simulink model "astrobee_control_sim"  (R2016b)
settings: configuration reference "cset" (kept outside this file)
PreLoadFcn:
  | astrobee_control_init;
  | astrobee_prep;
values from neighbouring files (symbols this model uses):
  astrobee_fsw_step_size = 0.016    [astrobee_control_init.m]    (also in astrobee_init.m)
  bus_cmc_msg_ic = Simulink.Bus.createMATLABStruct('cmc_msg')    [bus_init.m]
  bus_ctl_input_msg_ic = Simulink.Bus.createMATLABStruct('ctl_input_msg')    [bus_init.m]
undefined symbols (not defined in the file or in its folder): att_ki, att_kp, center_of_mass, cmc_mode_cmd, cmc_state_cmd_a, cmc_state_cmd_b, cmd_state_a, cmd_state_b, ctl_mode_cmd, current_time_nsec, current_time_sec, est_confidence, est_omega_B_ISS_B, est_P_B_ISS_ISS, est_quat_ISS2B, est_V_B_ISS_ISS, inertia_matrix, localization_mode_cmd, mass, omega_kd, pos_ki, pos_kp, speed_gain_cmd, tun_default_att_ki, tun_default_att_kp, tun_default_center_of_mass, tun_default_inertia_matrix, tun_default_mass, tun_default_omega_kd, tun_default_pos_ki, tun_default_pos_kp, tun_default_vel_kd, vel_kd
libraries: math_utils x3, cmc_command_and_mode_control x1, ctl_controller x1, env_environment_model_lib x1, fam_force_allocation_module_lib x1, simulink x1, veh_vehicle_model_lib x1
settings Model: Creator=mjmcinty  LastModifiedBy=jfusco1
settings ConfigSetRef: SourceLocation=Base Workspace

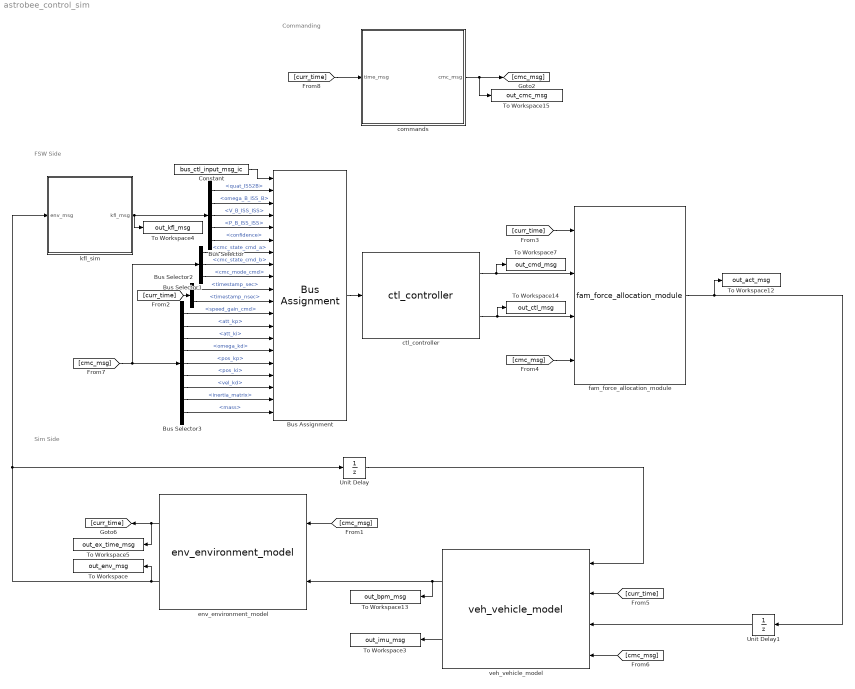
== system astrobee_control_sim ==
  note: FSW Side
  note: Sim Side
  note: Commanding
  Bus Assignment : BusAssignment  AssignedSignals=est_quat_ISS2B,est_omega_B_ISS_B,est_V_B_ISS_ISS,est_P_B_ISS_ISS,est_confidence,cmd_state_a,cmd_state_b,ctl_mode_cmd,current_time_sec,current_time_nsec,speed_gain_cmd,att_kp,att_ki,omega_kd,pos_kp,pos_ki,vel_kd,inertia_matrix,mass
  Bus Selector : BusSelector  OutputSignals=quat_ISS2B,omega_B_ISS_B,V_B_ISS_ISS,P_B_ISS_ISS,confidence
  Bus Selector1 : BusSelector  OutputSignals=cmc_state_cmd_a,cmc_state_cmd_b,cmc_mode_cmd
  Bus Selector2 : BusSelector  OutputSignals=timestamp_sec,timestamp_nsec
  Bus Selector3 : BusSelector  OutputSignals=speed_gain_cmd,att_kp,att_ki,omega_kd,pos_kp,pos_ki,vel_kd,inertia_matrix,mass
  Constant : Constant  Value=bus_ctl_input_msg_ic  OutDataTypeStr=Bus: ctl_input_msg
  To Workspace : ToWorkspace  VariableName=out_env_msg  SaveFormat=Timeseries  SampleTime=-1
  To Workspace12 : ToWorkspace  VariableName=out_act_msg  SaveFormat=Timeseries  SampleTime=-1
  To Workspace13 : ToWorkspace  VariableName=out_bpm_msg  SaveFormat=Timeseries  SampleTime=-1
  To Workspace14 : ToWorkspace  VariableName=out_ctl_msg  SaveFormat=Timeseries  SampleTime=-1
  To Workspace15 : ToWorkspace  VariableName=out_cmc_msg  SaveFormat=Timeseries  SampleTime=-1
  To Workspace3 : ToWorkspace  VariableName=out_imu_msg  SaveFormat=Timeseries  SampleTime=-1
  To Workspace4 : ToWorkspace  VariableName=out_kfl_msg  SaveFormat=Timeseries  SampleTime=-1
  To Workspace5 : ToWorkspace  VariableName=out_ex_time_msg  SaveFormat=Timeseries  SampleTime=-1
  To Workspace7 : ToWorkspace  VariableName=out_cmd_msg  SaveFormat=Timeseries  SampleTime=-1
  Unit Delay : UnitDelay  SampleTime=-1
  Unit Delay1 : UnitDelay  SampleTime=-1
  commands : Subsystem
  ctl_controller : ctl_controller/ctl_controller
  env_environment_model : env_environment_model_lib/env_environment_model  VariantControl=(default)
  fam_force_allocation_module : fam_force_allocation_module_lib/fam_force_allocation_module
  kfl_sim : Subsystem
  veh_vehicle_model : veh_vehicle_model_lib/veh_vehicle_model
  wires:
  [cmc_msg] -> fam_force_allocation_module/4
  env_environment_model/2 -> To Workspace/1, Unit Delay/1, kfl_sim/1(env_msg)
  ctl_controller/2 -> To Workspace14/1, fam_force_allocation_module/3
  ctl_controller/1 -> To Workspace7/1, fam_force_allocation_module/2
  [curr_time] -> fam_force_allocation_module/1
  commands/1(cmc_msg) -> To Workspace15/1, [cmc_msg]
  fam_force_allocation_module/1 -> To Workspace12/1, Unit Delay1/1
  [cmc_msg] -> env_environment_model/1
  [cmc_msg] -> veh_vehicle_model/4
  kfl_sim/1(kfl_msg) -> To Workspace4/1, Bus Selector/1
  veh_vehicle_model/1 -> To Workspace13/1, env_environment_model/2
  env_environment_model/1 -> To Workspace5/1, [curr_time]
  veh_vehicle_model/2 -> To Workspace3/1
  Unit Delay/1 -> veh_vehicle_model/1
  [curr_time] -> veh_vehicle_model/2
  [curr_time] -> commands/1(time_msg)
  Unit Delay1/1 -> veh_vehicle_model/3
  Bus Selector3/9 -> Bus Assignment/20  "<mass>"
  Bus Selector3/8 -> Bus Assignment/19  "<inertia_matrix>"
  Bus Selector3/7 -> Bus Assignment/18  "<vel_kd>"
  Bus Selector3/6 -> Bus Assignment/17  "<pos_ki>"
  Bus Selector3/5 -> Bus Assignment/16  "<pos_kp>"
  Bus Selector3/4 -> Bus Assignment/15  "<omega_kd>"
  Bus Selector3/3 -> Bus Assignment/14  "<att_ki>"
  Bus Selector3/2 -> Bus Assignment/13  "<att_kp>"
  Bus Selector3/1 -> Bus Assignment/12  "<speed_gain_cmd>"
  Bus Selector2/2 -> Bus Assignment/11  "<timestamp_nsec>"
  Bus Selector2/1 -> Bus Assignment/10  "<timestamp_sec>"
  [curr_time] -> Bus Selector2/1
  Bus Selector1/3 -> Bus Assignment/9  "<cmc_mode_cmd>"
  Bus Selector1/2 -> Bus Assignment/8  "<cmc_state_cmd_b>"
  Bus Selector1/1 -> Bus Assignment/7  "<cmc_state_cmd_a>"
  Bus Selector/5 -> Bus Assignment/6  "<confidence>"
  Bus Selector/4 -> Bus Assignment/5  "<P_B_ISS_ISS>"
  Bus Selector/1 -> Bus Assignment/2  "<quat_ISS2B>"
  Bus Selector/3 -> Bus Assignment/4  "<V_B_ISS_ISS>"
  Bus Selector/2 -> Bus Assignment/3  "<omega_B_ISS_B>"
  Constant/1 -> Bus Assignment/1
  [cmc_msg] -> Bus Selector1/1, Bus Selector3/1
  Bus Assignment/1 -> ctl_controller/1

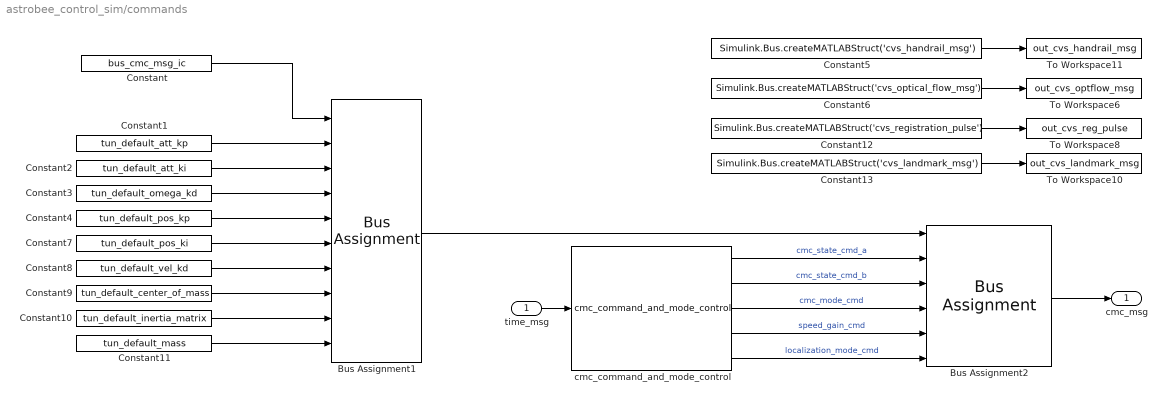
== system astrobee_control_sim/commands ==
  time_msg : Inport
  Bus Assignment1 : BusAssignment  AssignedSignals=att_kp,att_ki,omega_kd,pos_kp,pos_ki,vel_kd,center_of_mass,inertia_matrix,mass
  Bus Assignment2 : BusAssignment  AssignedSignals=cmc_state_cmd_a,cmc_state_cmd_b,cmc_mode_cmd,speed_gain_cmd,localization_mode_cmd
  Constant : Constant  Value=bus_cmc_msg_ic  OutDataTypeStr=Bus: cmc_msg
  Constant1 : Constant  Value=tun_default_att_kp
  Constant10 : Constant  Value=tun_default_inertia_matrix
  Constant11 : Constant  Value=tun_default_mass
  Constant12 : Constant  Value=Simulink.Bus.createMATLABStruct('cvs_registration_pulse')  OutDataTypeStr=Bus: cvs_registration_pulse
  Constant13 : Constant  Value=Simulink.Bus.createMATLABStruct('cvs_landmark_msg')  OutDataTypeStr=Bus: cvs_landmark_msg
  Constant2 : Constant  Value=tun_default_att_ki
  Constant3 : Constant  Value=tun_default_omega_kd
  Constant4 : Constant  Value=tun_default_pos_kp
  Constant5 : Constant  Value=Simulink.Bus.createMATLABStruct('cvs_handrail_msg')  OutDataTypeStr=Bus: cvs_handrail_msg
  Constant6 : Constant  Value=Simulink.Bus.createMATLABStruct('cvs_optical_flow_msg')  OutDataTypeStr=Bus: cvs_optical_flow_msg
  Constant7 : Constant  Value=tun_default_pos_ki
  Constant8 : Constant  Value=tun_default_vel_kd
  Constant9 : Constant  Value=tun_default_center_of_mass
  To Workspace10 : ToWorkspace  VariableName=out_cvs_landmark_msg  SaveFormat=Timeseries  SampleTime=-1
  To Workspace11 : ToWorkspace  VariableName=out_cvs_handrail_msg  SaveFormat=Timeseries  SampleTime=-1
  To Workspace6 : ToWorkspace  VariableName=out_cvs_optflow_msg  SaveFormat=Timeseries  SampleTime=-1
  To Workspace8 : ToWorkspace  VariableName=out_cvs_reg_pulse  SaveFormat=Timeseries  SampleTime=-1
  cmc_command_and_mode_control : cmc_command_and_mode_control/cmc_command_and_mode_control
  cmc_msg : Outport  OutDataTypeStr=Bus: cmc_msg
  wires:
  Constant3/1 -> Bus Assignment1/4
  Constant4/1 -> Bus Assignment1/5
  Constant2/1 -> Bus Assignment1/3
  Constant7/1 -> Bus Assignment1/6
  Constant1/1 -> Bus Assignment1/2
  Constant8/1 -> Bus Assignment1/7
  Constant9/1 -> Bus Assignment1/8
  Constant10/1 -> Bus Assignment1/9
  Constant11/1 -> Bus Assignment1/10
  Constant/1 -> Bus Assignment1/1
  cmc_command_and_mode_control/4 -> Bus Assignment2/5  "speed_gain_cmd"
  cmc_command_and_mode_control/5 -> Bus Assignment2/6  "localization_mode_cmd"
  time_msg/1 -> cmc_command_and_mode_control/1
  cmc_command_and_mode_control/2 -> Bus Assignment2/3  "cmc_state_cmd_b"
  cmc_command_and_mode_control/3 -> Bus Assignment2/4  "cmc_mode_cmd"
  cmc_command_and_mode_control/1 -> Bus Assignment2/2  "cmc_state_cmd_a"
  Bus Assignment2/1 -> cmc_msg/1
  Bus Assignment1/1 -> Bus Assignment2/1
  Constant5/1 -> To Workspace11/1
  Constant6/1 -> To Workspace6/1
  Constant12/1 -> To Workspace8/1
  Constant13/1 -> To Workspace10/1

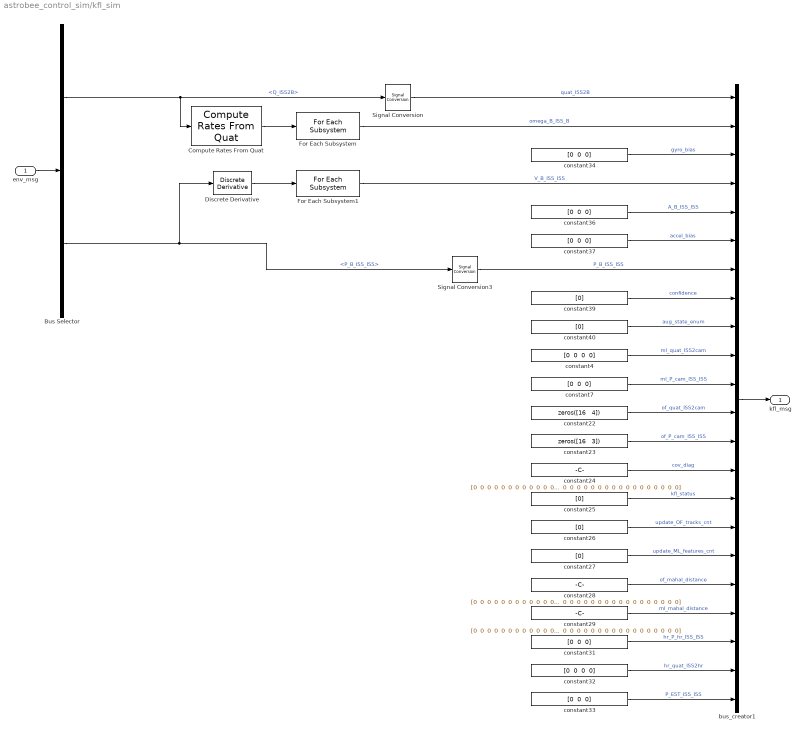
== system astrobee_control_sim/kfl_sim ==
  env_msg : Inport  OutDataTypeStr=Bus: env_msg
  Bus Selector : BusSelector  OutputSignals=Q_ISS2B,P_B_ISS_ISS
  Compute Rates From Quat : math_utils/Compute Rates From Quat  SystemSampleTime=-1
  Discrete Derivative : simulink/Discrete/Discrete Derivative  gainval=1.0  ICPrevScaledInput=0.0  OutMin=[]  OutMax=[]  OutDataType=fixdt(1, 16)  OutScaling=2^-10  DoSatur=off
  For Each Subsystem : math_utils/For Each Subsystem  T=astrobee_fsw_step_size  omega=tun_truth_q_omega_filt_cutoff_freq  filt_enable=tun_truth_q_omega_filt_enable
  For Each Subsystem1 : math_utils/For Each Subsystem  T=astrobee_fsw_step_size  omega=tun_truth_velocity_filt_cutoff_freq  filt_enable=tun_truth_velocity_filt_enable
  Signal Conversion : SignalConversion  OverrideOpt=off
  Signal Conversion3 : SignalConversion  OverrideOpt=off
  bus_creator1 : BusCreator  Inputs=22  OutDataTypeStr=Bus: kfl_msg  NonVirtualBus=on
  constant22 : Constant  Value="zeros([16   4])"  OutDataTypeStr=single
  constant23 : Constant  Value="zeros([16   3])"  OutDataTypeStr=single
  constant24 : Constant  Value="[0  0  0  0  0  0  0  0  0  0  0  0  0  0  0  0  0  0  0  0  0  0  0  0  0  0  0  0  0  0  0  0  0  0  0  0  0  0  0  0  0  0  0  0  0  0  0  0  0  0  0  0  0  0  0  0  0  0  0  0  0  0  0  0  0  0  0  0  0  0  0  0  0  0  0  0  0  0  0  0  0  0  0  0  0  0  0  0  0  0  0  0  0  0  0  0  0  0  0  0  0  0  0  0  0  0  0  0  0  0  0  0  0  0  0  0  0]"  OutDataTypeStr=ase_cov_datatype
  constant25 : Constant  Value=[0]  OutDataTypeStr=uint16
  constant26 : Constant  Value=[0]  OutDataTypeStr=uint8
  constant27 : Constant  Value=[0]  OutDataTypeStr=uint8
  constant28 : Constant  Value="[0  0  0  0  0  0  0  0  0  0  0  0  0  0  0  0  0  0  0  0  0  0  0  0  0  0  0  0  0  0  0  0  0  0  0  0  0  0  0  0  0  0  0  0  0  0  0  0  0  0]"  OutDataTypeStr=double
  constant29 : Constant  Value="[0  0  0  0  0  0  0  0  0  0  0  0  0  0  0  0  0  0  0  0  0  0  0  0  0  0  0  0  0  0  0  0  0  0  0  0  0  0  0  0  0  0  0  0  0  0  0  0  0  0]"  OutDataTypeStr=double
  constant{7,31,33..34,36..37} (6 alike) : Constant  Value="[0  0  0]"  OutDataTypeStr=single
  constant32 : Constant  Value="[0  0  0  0]"  OutDataTypeStr=single
  constant39 : Constant  Value=[0]  OutDataTypeStr=uint8
  constant4 : Constant  Value="[0  0  0  0]"  OutDataTypeStr=single
  constant40 : Constant  Value=[0]  OutDataTypeStr=uint32
  kfl_msg : Outport
  wires:
  Discrete Derivative/1 -> For Each Subsystem1/1
  Compute Rates From Quat/1 -> For Each Subsystem/1
  bus_creator1/1 -> kfl_msg/1
  constant33/1 -> bus_creator1/22  "P_EST_ISS_ISS"
  constant32/1 -> bus_creator1/21  "hr_quat_ISS2hr"
  constant31/1 -> bus_creator1/20  "hr_P_hr_ISS_ISS"
  constant29/1 -> bus_creator1/19  "ml_mahal_distance"
  constant28/1 -> bus_creator1/18  "of_mahal_distance"
  constant27/1 -> bus_creator1/17  "update_ML_features_cnt"
  constant26/1 -> bus_creator1/16  "update_OF_tracks_cnt"
  constant25/1 -> bus_creator1/15  "kfl_status"
  constant24/1 -> bus_creator1/14  "cov_diag"
  constant23/1 -> bus_creator1/13  "of_P_cam_ISS_ISS"
  constant22/1 -> bus_creator1/12  "of_quat_ISS2cam"
  constant7/1 -> bus_creator1/11  "ml_P_cam_ISS_ISS"
  constant4/1 -> bus_creator1/10  "ml_quat_ISS2cam"
  constant40/1 -> bus_creator1/9  "aug_state_enum"
  constant39/1 -> bus_creator1/8  "confidence"
  Signal Conversion3/1 -> bus_creator1/7  "P_B_ISS_ISS"
  constant37/1 -> bus_creator1/6  "accel_bias"
  constant36/1 -> bus_creator1/5  "A_B_ISS_ISS"
  For Each Subsystem1/1 -> bus_creator1/4  "V_B_ISS_ISS"
  constant34/1 -> bus_creator1/3  "gyro_bias"
  For Each Subsystem/1 -> bus_creator1/2  "omega_B_ISS_B"
  Signal Conversion/1 -> bus_creator1/1  "quat_ISS2B"
  env_msg/1 -> Bus Selector/1
  Bus Selector/1 -> Compute Rates From Quat/1, Signal Conversion/1  "<Q_ISS2B>"
  Bus Selector/2 -> Signal Conversion3/1, Discrete Derivative/1  "<P_B_ISS_ISS>"
